simulink model "C_LQG"  (R2020b)
settings: Solver=VariableStepAuto  StartTime=0.0  StopTime=30  RelTol=1e-3
values from neighbouring files (symbols this model uses):
  sysE = ss(tf(48*(Kt/Ra)))    [C_Hinf.m]
  sysM = ss(tf(Ra,[Ra*J Ke*Kt+Ra*B 0]))    [C_Hinf.m]
undefined symbols (not defined in the file or in its folder): K1, sysKF
settings Model: Creator=andre  LastModifiedBy=andre

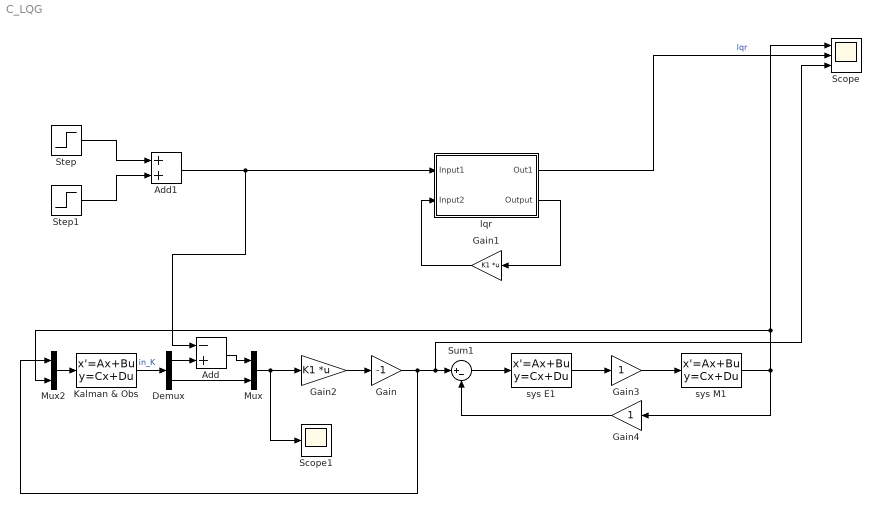
== system C_LQG ==
  Add : Sum  Inputs=-+
  Add1 : Sum
  Demux : Demux  Outputs=2
  Gain : Gain  Gain=-1
  Gain1 : Gain  Gain=K1  Multiplication=Matrix(K*u) (u vector)
  Gain2 : Gain  Gain=K1  Multiplication=Matrix(K*u) (u vector)
  Gain3 : Gain
  Gain4 : Gain
  Kalman & Obs : StateSpace  A=sysKF.A  B=sysKF.B  C=sysKF.C  D=sysKF.D  InitialCondition=0
  Mux : Mux  Inputs=2
  Mux2 : Mux  Inputs=2
  Scope : Scope  NumInputPorts=3
  Scope1 : Scope
  Step : Step  Time=0  After=5  SampleTime=0
  Step1 : Step  Time=5  After=-5  SampleTime=0
  Sum1 : Sum  Inputs=|+-
  lqr : Subsystem
  sys E1 : StateSpace  A=sysE.A  B=sysE.B  C=sysE.C  D=sysE.D  InitialCondition=0
  sys M1 : StateSpace  A=sysM.A  B=sysM.B  C=sysM.C  D=sysM.D  InitialCondition=0
  wires:
  lqr/2(Output) -> Gain1/1
  Gain1/1 -> lqr/2(Input2)
  lqr/1(Out1) -> Scope/2  "lqr"
  Gain2/1 -> Gain/1
  Mux2/1 -> Kalman & Obs/1
  sys M1/1 -> Mux2/2, Scope/1, Gain4/1
  Gain4/1 -> Sum1/2
  Gain3/1 -> sys M1/1
  sys E1/1 -> Gain3/1
  Sum1/1 -> sys E1/1
  Kalman & Obs/1 -> Demux/1  "in_K"
  Mux/1 -> Scope1/1, Gain2/1
  Demux/1 -> Add/2
  Add1/1 -> Add/1, lqr/1(Input1)
  Demux/2 -> Mux/2
  Add/1 -> Mux/1
  Gain/1 -> Scope/3, Sum1/1, Mux2/1
  Step/1 -> Add1/1
  Step1/1 -> Add1/2

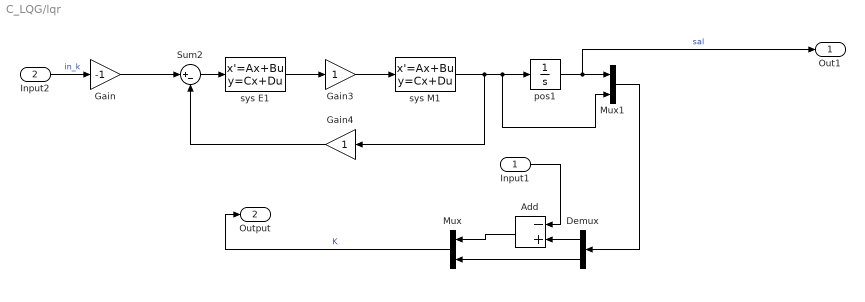
== system C_LQG/lqr ==
  Input1 : Inport
  Input2 : Inport  Port=2
  Add : Sum  Inputs=-+
  Demux : Demux  Outputs=2
  Gain : Gain  Gain=-1
  Gain3 : Gain
  Gain4 : Gain
  Mux : Mux  Inputs=2
  Mux1 : Mux  Inputs=2
  Sum2 : Sum  Inputs=|+-
  pos1 : Integrator
  sys E1 : StateSpace  A=sysE.A  B=sysE.B  C=sysE.C  D=sysE.D  InitialCondition=0
  sys M1 : StateSpace  A=sysM.A  B=sysM.B  C=sysM.C  D=sysM.D  InitialCondition=0
  Out1 : Outport
  Output : Outport  Port=2
  wires:
  sys E1/1 -> Gain3/1
  sys M1/1 -> Mux1/2, pos1/1, Gain4/1
  Gain4/1 -> Sum2/2
  Mux/1 -> Output/1  "K"
  Demux/1 -> Add/2
  Gain3/1 -> sys M1/1
  Sum2/1 -> sys E1/1
  Add/1 -> Mux/1
  pos1/1 -> Out1/1, Mux1/1  "sal"
  Mux1/1 -> Demux/1
  Input1/1 -> Add/1
  Demux/2 -> Mux/2
  Gain/1 -> Sum2/1
  Input2/1 -> Gain/1  "in_k"
